simulink model "project1_demo"  (R2023b)
settings: Solver=VariableStepAuto  StartTime=0.0  StopTime=25  RelTol=1e-3
model workspace (MAT data in the model file):
  J = Simulink.Parameter
  J.DataType = 'auto'
  J.Complexity = 'real'
  J.Dimensions = [0 0]
values from neighbouring files (symbols this model uses):
  b = B(x)    [Project_1.m]
  j = J1(y)    [Project_1.m]
  p_0 = 0    [Project_1.m]
  T = AT(w)    [Project_1.m]
  w_0 = W_0(z)    [Project_1.m]    (also in Week1_WorkingCode.m = 1)
settings Model: Creator=Christina  LastModifiedBy=nakro

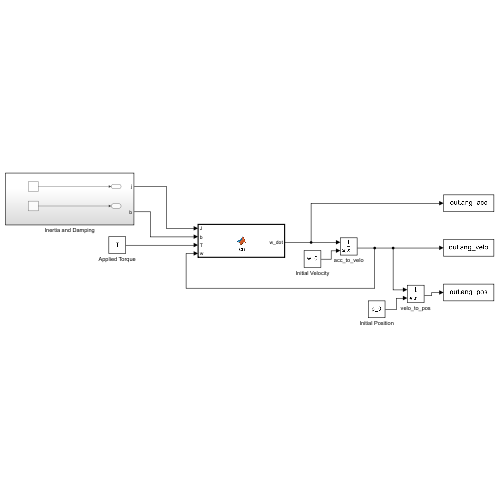
[thumbnail: Simulink's stored preview of the top-level diagram]
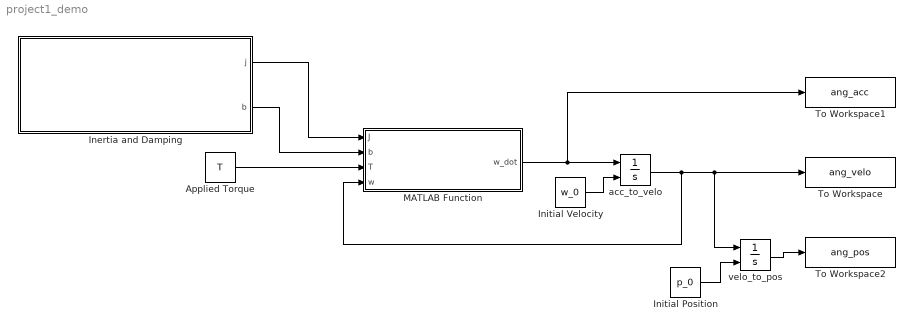
== system project1_demo ==
  Applied Torque : Constant  Value=T
  Inertia and Damping : Subsystem
  Initial Position : Constant  Value=p_0
  Initial Velocity : Constant  Value=w_0
  MATLAB Function : MATLAB Function  TreatAsAtomicUnit=on
  To Workspace : ToWorkspace  VariableName=ang_velo  SaveFormat=Timeseries  SampleTime=-1
  To Workspace1 : ToWorkspace  VariableName=ang_acc  SaveFormat=Timeseries  SampleTime=-1
  To Workspace2 : ToWorkspace  VariableName=ang_pos  SaveFormat=Timeseries  SampleTime=-1
  acc_to_velo : Integrator  InitialConditionSource=external
  velo_to_pos : Integrator  InitialConditionSource=external
  wires:
  Applied Torque/1 -> MATLAB Function/3(T)
  MATLAB Function/1(w_dot) -> To Workspace1/1, acc_to_velo/1
  acc_to_velo/1 -> velo_to_pos/1, To Workspace/1, MATLAB Function/4(w)
  Initial Velocity/1 -> acc_to_velo/2
  Inertia and Damping/1(j) -> MATLAB Function/1(J)
  Inertia and Damping/2(b) -> MATLAB Function/2(b)
  velo_to_pos/1 -> To Workspace2/1
  Initial Position/1 -> velo_to_pos/2

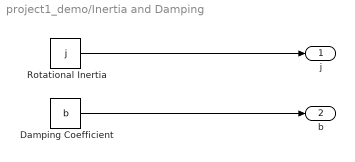
== system project1_demo/Inertia and Damping ==
  Damping Coefficient : Constant  Value=b
  Rotational Inertia : Constant  Value=j
  j : Outport
  b : Outport  Port=2
  wires:
  Rotational Inertia/1 -> j/1
  Damping Coefficient/1 -> b/1

== matlab function project1_demo/MATLAB Function ==
  data: J input; b input; w_dot output; T input; w input
function w_dot = fcn(J, b, T, w)

w_dot = (1/J)*(T-(b*w));

end
